simulink model "f_oscillateur"  (R2015a)
settings: Solver=ode45  StartTime=0.0  StopTime=0.1  MaxStep=1e-6  MinStep=1e-10  RelTol=1e-3
values from neighbouring files (symbols this model uses):
  denC = [R*C 1]    [fp_oscillateur.m]    (also in tp_oscillateur.m)
  denG = [1/(2*pi*f0) 1]    [fp_oscillateur.m]    (also in tp_oscillateur.m)
  K = 1e-6    (= 1e-06)    [BodeTest.m]    (also in fp_oscillateur.m = 0.0001; test_multiple.m = linspace(0,1e-4,50); tp_oscillateur.m = 0.0001)
  numC = 1    [fp_oscillateur.m]    (also in tp_oscillateur.m)
  numG = A0    (= 100000)    [fp_oscillateur.m]    (also in tp_oscillateur.m)
settings Model: Creator=mserrari  LastModifiedBy=mserrari
settings SolverCC: InitialStep=1e-8

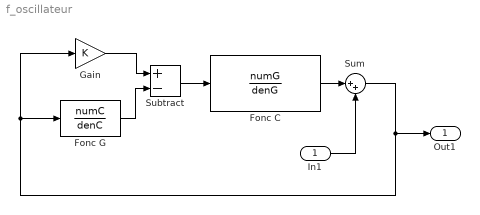
== system f_oscillateur ==
  In1 : Inport
  Fonc C : TransferFcn  Numerator=numG  Denominator=denG
  Fonc G : TransferFcn  Numerator=numC  Denominator=denC
  Gain : Gain  Gain=K
  Subtract : Sum  Inputs=+-
  Sum : Sum  Inputs=|++
  Out1 : Outport
  wires:
  Fonc G/1 -> Subtract/2
  Gain/1 -> Subtract/1
  Subtract/1 -> Fonc C/1
  Fonc C/1 -> Sum/1
  Sum/1 -> Out1/1, Gain/1, Fonc G/1
  In1/1 -> Sum/2
